simulink model "joy_send"  (R2016b)
settings: Solver=VariableStepAuto  StartTime=0.0  StopTime=inf  RelTol=1e-3
libraries: dspnetwork x2
settings Model: Creator=supak  LastModifiedBy=supak

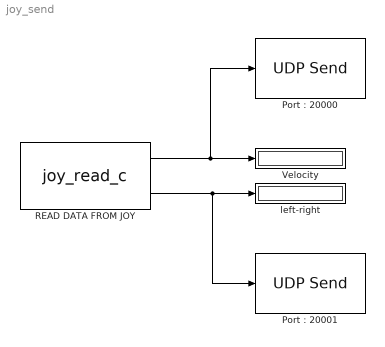
== system joy_send ==
  "Port : 20000" : dspnetwork/UDP Send  remoteURL='192.168.1.118'  remotePort=20000  localURL='0.0.0.0'  localPortSource=Automatically determine  localPort=-1  sampletime=-1  blockPlatform=HOST  separateLengthPort=0
  "Port : 20001" : dspnetwork/UDP Send  remoteURL='192.168.1.118'  remotePort=20001  localURL='0.0.0.0'  localPortSource=Automatically determine  localPort=-1  sampletime=-1  blockPlatform=HOST  separateLengthPort=0
  READ DATA FROM JOY : S-Function  FunctionName=joy_read_c  SFunctionModules='joy_read_c'  SFunctionDeploymentMode=off  EnableBusSupport=off
  Velocity : Display
  left-right : Display
  wires:
  READ DATA FROM JOY/1 -> "Port : 20000"/1, Velocity/1
  READ DATA FROM JOY/2 -> "Port : 20001"/1, left-right/1
